simulink model "HCO"  (R2023b)
settings: Solver=VariableStepAuto  StartTime=0.0  StopTime=1  RelTol=1e-3
libraries: simulink x2
settings Model: Creator=Dayan-pc  LastModifiedBy=Dayan-pc
settings OptimizationCC: ReuseModelBlockBuffer=off

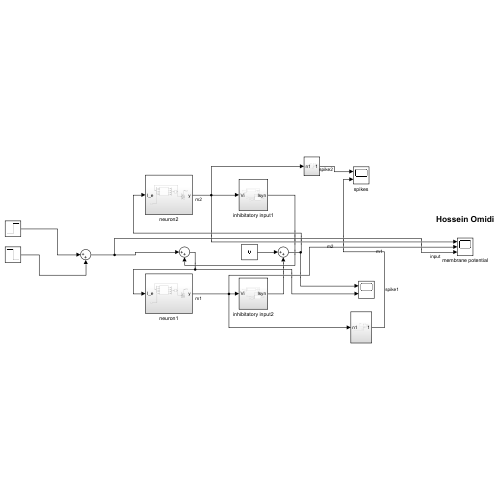
[thumbnail: Simulink's stored preview of the top-level diagram]
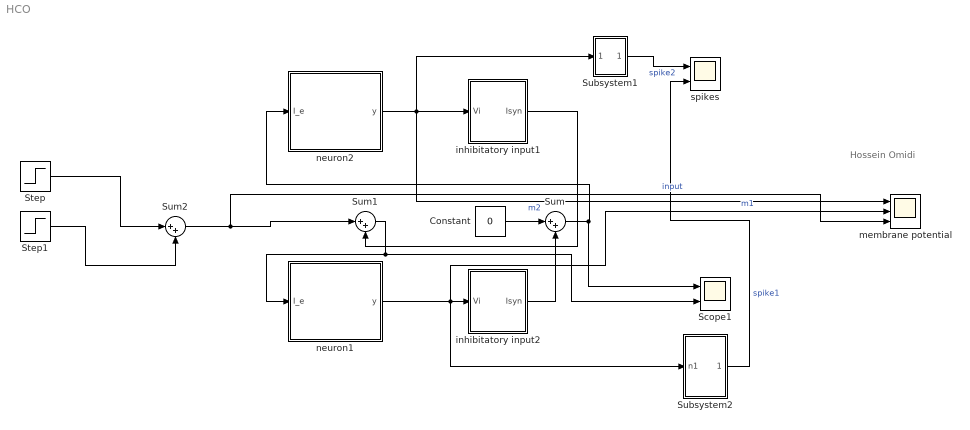
== system HCO ==
  note: Hossein Omidi
  Constant : Constant  Value=0
  Scope1 : Scope  NumInputPorts=2
  Step : Step  Time=.3  After=10  SampleTime=0
  Step1 : Step  Time=.31  After=-10  SampleTime=0
  Subsystem1 : Subsystem
  Subsystem2 : Subsystem
  Sum : Sum  Inputs=|++
  Sum1 : Sum  Inputs=|++
  Sum2 : Sum  Inputs=|++
  inhibitatory input1 : Subsystem
  inhibitatory input2 : Subsystem
  membrane potential : Scope  NumInputPorts=3
  neuron1 : Subsystem
  neuron2 : Subsystem
  spikes : Scope  NumInputPorts=2
  wires:
  neuron2/1(y) -> Subsystem1/1(n1), membrane potential/1, inhibitatory input1/1(Vi)  "m2"
  neuron1/1(y) -> Subsystem2/1(n1), membrane potential/2, inhibitatory input2/1(Vi)  "m1"
  inhibitatory input2/1(Isyn) -> Sum/2
  Sum/1 -> Scope1/1, neuron2/1(I_e)
  Sum1/1 -> Scope1/2, neuron1/1(I_e)
  inhibitatory input1/1(Isyn) -> Sum1/2
  Sum2/1 -> membrane potential/3, Sum1/1  "input"
  Step1/1 -> Sum2/2
  Step/1 -> Sum2/1
  Constant/1 -> Sum/1
  Subsystem1/1(Out1) -> spikes/1  "spike2"
  Subsystem2/1(Out1) -> spikes/2  "spike1"

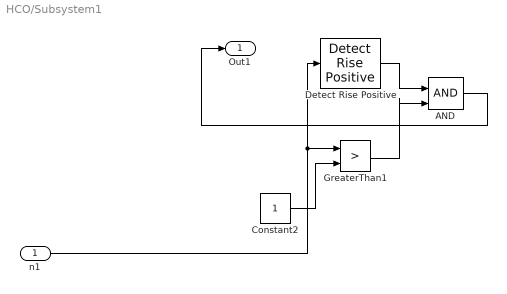
== system HCO/Subsystem1 ==
  n1 : Inport
  AND : Logic  IconShape=distinctive  AllPortsSameDT=off  OutDataTypeStr=boolean
  Constant2 : Constant
  Detect Rise Positive : simulink/Logic and Bit Operations/Detect Rise Positive  vinit=0  OutDataTypeStr=boolean
  GreaterThan1 : RelationalOperator  Operator=>  OutDataTypeStr=boolean  RndMeth=Simplest  InputSameDT=off
  Out1 : Outport
  wires:
  GreaterThan1/1 -> AND/2
  Detect Rise Positive/1 -> AND/1
  Constant2/1 -> GreaterThan1/2
  n1/1 -> GreaterThan1/1, Detect Rise Positive/1
  AND/1 -> Out1/1

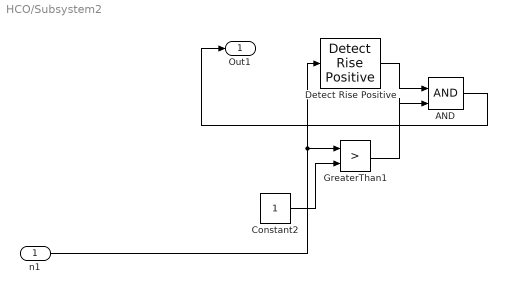
== system HCO/Subsystem2 ==
  n1 : Inport
  AND : Logic  IconShape=distinctive  AllPortsSameDT=off  OutDataTypeStr=boolean
  Constant2 : Constant
  Detect Rise Positive : simulink/Logic and Bit Operations/Detect Rise Positive  vinit=0  OutDataTypeStr=boolean
  GreaterThan1 : RelationalOperator  Operator=>  OutDataTypeStr=boolean  RndMeth=Simplest  InputSameDT=off
  Out1 : Outport
  wires:
  AND/1 -> Out1/1
  n1/1 -> Detect Rise Positive/1, GreaterThan1/1
  Constant2/1 -> GreaterThan1/2
  Detect Rise Positive/1 -> AND/1
  GreaterThan1/1 -> AND/2

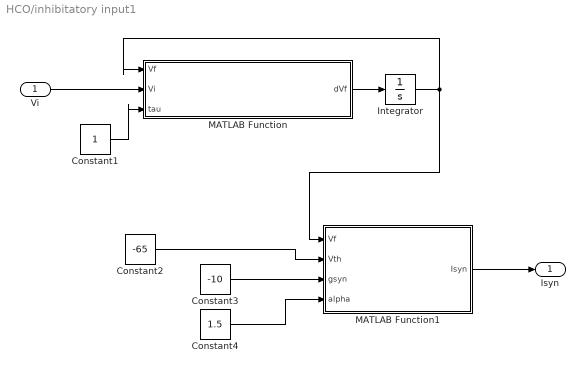
== system HCO/inhibitatory input1 ==
  Vi : Inport
  Constant1 : Constant
  Constant2 : Constant  Value=-65
  Constant3 : Constant  Value=-10
  Constant4 : Constant  Value=1.5
  Integrator : Integrator
  MATLAB Function : MATLAB Function  TreatAsAtomicUnit=on
  MATLAB Function1 : MATLAB Function  TreatAsAtomicUnit=on
  Isyn : Outport
  wires:
  MATLAB Function1/1(Isyn) -> Isyn/1
  Constant1/1 -> MATLAB Function/3(tau)
  Constant4/1 -> MATLAB Function1/4(alpha)
  MATLAB Function/1(dVf) -> Integrator/1
  Integrator/1 -> MATLAB Function1/1(Vf), MATLAB Function/1(Vf)
  Vi/1 -> MATLAB Function/2(Vi)
  Constant3/1 -> MATLAB Function1/3(gsyn)
  Constant2/1 -> MATLAB Function1/2(Vth)

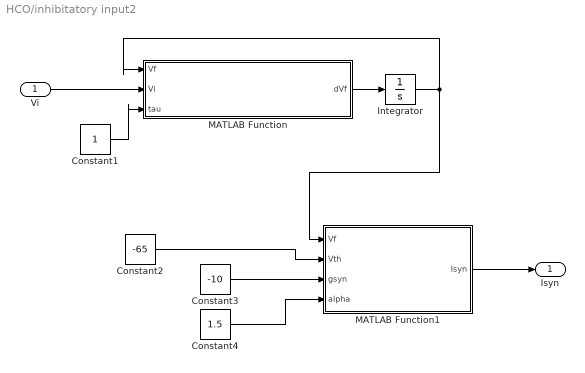
== system HCO/inhibitatory input2 ==
  Vi : Inport
  Constant1 : Constant
  Constant2 : Constant  Value=-65
  Constant3 : Constant  Value=-10
  Constant4 : Constant  Value=1.5
  Integrator : Integrator
  MATLAB Function : MATLAB Function  TreatAsAtomicUnit=on
  MATLAB Function1 : MATLAB Function  TreatAsAtomicUnit=on
  Isyn : Outport
  wires:
  Constant2/1 -> MATLAB Function1/2(Vth)
  Constant3/1 -> MATLAB Function1/3(gsyn)
  Vi/1 -> MATLAB Function/2(Vi)
  Integrator/1 -> MATLAB Function/1(Vf), MATLAB Function1/1(Vf)
  MATLAB Function/1(dVf) -> Integrator/1
  Constant4/1 -> MATLAB Function1/4(alpha)
  Constant1/1 -> MATLAB Function/3(tau)
  MATLAB Function1/1(Isyn) -> Isyn/1

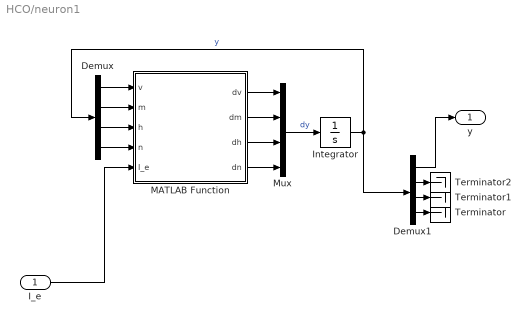
== system HCO/neuron1 ==
  I_e : Inport
  Demux : Demux
  Demux1 : Demux
  Integrator : Integrator  InitialCondition=[-65; 0.05; 0.60; 0.32]
  MATLAB Function : MATLAB Function  TreatAsAtomicUnit=on
  Mux : Mux
  Terminator : Terminator
  Terminator1 : Terminator
  Terminator2 : Terminator
  y : Outport
  wires:
  Demux1/1 -> y/1
  Demux1/2 -> Terminator2/1
  Demux1/3 -> Terminator1/1
  Demux1/4 -> Terminator/1
  I_e/1 -> MATLAB Function/5(I_e)
  MATLAB Function/2(dm) -> Mux/2
  Demux/4 -> MATLAB Function/4(n)
  Demux/2 -> MATLAB Function/2(m)
  Demux/3 -> MATLAB Function/3(h)
  Integrator/1 -> Demux1/1, Demux/1  "y"
  MATLAB Function/4(dn) -> Mux/4
  MATLAB Function/3(dh) -> Mux/3
  Demux/1 -> MATLAB Function/1(v)
  Mux/1 -> Integrator/1  "dy"
  MATLAB Function/1(dv) -> Mux/1

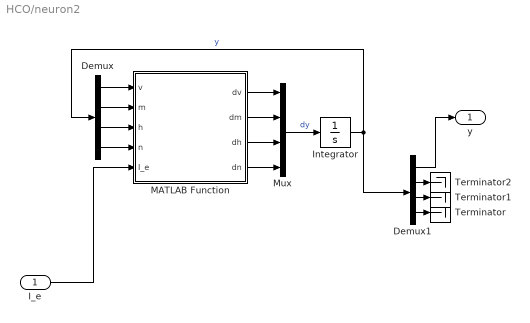
== system HCO/neuron2 ==
  I_e : Inport
  Demux : Demux
  Demux1 : Demux
  Integrator : Integrator  InitialCondition=[-65; 0.05; 0.60; 0.32]
  MATLAB Function : MATLAB Function  TreatAsAtomicUnit=on
  Mux : Mux
  Terminator : Terminator
  Terminator1 : Terminator
  Terminator2 : Terminator
  y : Outport
  wires:
  MATLAB Function/1(dv) -> Mux/1
  Mux/1 -> Integrator/1  "dy"
  Demux/1 -> MATLAB Function/1(v)
  MATLAB Function/3(dh) -> Mux/3
  MATLAB Function/4(dn) -> Mux/4
  Integrator/1 -> Demux/1, Demux1/1  "y"
  Demux/3 -> MATLAB Function/3(h)
  Demux/2 -> MATLAB Function/2(m)
  Demux/4 -> MATLAB Function/4(n)
  MATLAB Function/2(dm) -> Mux/2
  I_e/1 -> MATLAB Function/5(I_e)
  Demux1/4 -> Terminator/1
  Demux1/3 -> Terminator1/1
  Demux1/2 -> Terminator2/1
  Demux1/1 -> y/1

== matlab function HCO/inhibitatory input2/MATLAB Function ==
  data: Vf input; dVf output; Vi input; tau input
function dVf = synapse_filter_deriv(Vf, Vi, tau)
% ODE for the synaptic low-pass filter state Vf
% tau * dVf/dt = Vpre - Vf  ->  dVf/dt = (Vpre - Vf)/tau
% Inputs:
%   Vf   - current filter state (mV)
%   Vpre - presynaptic membrane voltage (mV)
%   tau  - filter time constant (ms, >0)
% Output:
%   dVf  - time derivative of Vf (mV/ms)

% numeric safety

dVf = 1000*(Vi - Vf) / tau;
end

== matlab function HCO/neuron2/MATLAB Function ==
  data: v input; dv output; m input; h input; n input; I_e input; dm output; dh output; dn output
function [dv, dm, dh, dn] = hh_block(v, m, h, n, I_e)
% HH ODEs for Simulink MATLAB Function block
% Inputs: v,m,h,n (states), I_e total injected current (uA/cm^2)
% Outputs: dv,dm,dh,dn (state derivatives)

    % Params
    C_m = 1.0; gNa = 120.0; gK = 36.0; gL = 0.3;
    ENa = 50.0; EK = -77.0; EL = -54.387;

    % Safe division
    am_num = 0.1 * (v + 40.0);
    am_den = 1.0 - exp(-(v + 40.0)/10.0);
    %if abs(am_den) < epsd, am_den = sign(am_den)*epsd + (am_den==0)*epsd; end
    alpha_m = am_num / am_den;

    beta_m = 4.0 * exp(-(v + 65.0)/18.0);
    alpha_h = 0.07 * exp(-(v + 65.0)/20.0);
    beta_h  = 1.0 / (1.0 + exp(-(v + 35.0)/10.0));

    an_num = 0.01 * (v + 55.0);
    an_den = 1.0 - exp(-(v + 55.0)/10.0);
    %if abs(an_den) < epsd, an_den = sign(an_den)*epsd + (an_den==0)*epsd; end
    alpha_n = an_num / an_den;

    beta_n = 0.125 * exp(-(v + 65.0)/80.0);

    % x_inf and tau
    denom_m = alpha_m + beta_m; 
    denom_h = alpha_h + beta_h; 
    denom_n = alpha_n + beta_n;

    m_inf = alpha_m / denom_m; tau_m = 1.0 / denom_m;
    h_inf = alpha_h / denom_h; tau_h = 1.0 / denom_h;
    n_inf = alpha_n / denom_n; tau_n = 1.0 / denom_n;

    % Currents
    I_Na = gNa * (m^3) * h * (v - ENa);
    I_K  = gK  * (n^4) * (v - EK);
    I_L  = gL  * (v - EL);

    % ODEs
    dv = 1000*(-I_L - I_Na - I_K + I_e) / C_m;
    dm = 1000*(m_inf - m) / tau_m;
    dh = 1000*(h_inf - h) / tau_h;
    dn = 1000*(n_inf - n) / tau_n;
end

== matlab function HCO/inhibitatory input2/MATLAB Function1 ==
  data: Vf input; Isyn output; Vth input; gsyn input; alpha input
function Isyn = synapse_current(Vf, Vth, gsyn, alpha)
% Current-based synapse (paper's model)
% Isyn = gsyn / (1 + exp(-alpha*(Vf - Vth)))
% Inputs:
%   Vf    - filtered presynaptic voltage (mV)
%   Vth   - threshold (mV)
%   gsyn  - synaptic strength (uA/cm^2). >0 excitatory, <0 inhibitory
%   alpha - sigmoid slope (>0)
% Output:
%   Isyn  - synaptic current to inject into postsynaptic neuron (uA/cm^2)



% Synapse nonlinearity (paper)
s = Vf - Vth;                % onto neuron 2
Isyn = gsyn / (1 + exp(-alpha * s));
end

== matlab function HCO/neuron1/MATLAB Function ==
  data: v input; dv output; m input; h input; n input; I_e input; dm output; dh output; dn output
function [dv, dm, dh, dn] = hh_block(v, m, h, n, I_e)
% HH ODEs for Simulink MATLAB Function block
% Inputs: v,m,h,n (states), I_e total injected current (uA/cm^2)
% Outputs: dv,dm,dh,dn (state derivatives)

    % Params
    C_m = 1.0; gNa = 120.0; gK = 36.0; gL = 0.3;
    ENa = 50.0; EK = -77.0; EL = -54.387;

    % Safe division
    am_num = 0.1 * (v + 40.0);
    am_den = 1.0 - exp(-(v + 40.0)/10.0);
    %if abs(am_den) < epsd, am_den = sign(am_den)*epsd + (am_den==0)*epsd; end
    alpha_m = am_num / am_den;

    beta_m = 4.0 * exp(-(v + 65.0)/18.0);
    alpha_h = 0.07 * exp(-(v + 65.0)/20.0);
    beta_h  = 1.0 / (1.0 + exp(-(v + 35.0)/10.0));

    an_num = 0.01 * (v + 55.0);
    an_den = 1.0 - exp(-(v + 55.0)/10.0);
    %if abs(an_den) < epsd, an_den = sign(an_den)*epsd + (an_den==0)*epsd; end
    alpha_n = an_num / an_den;

    beta_n = 0.125 * exp(-(v + 65.0)/80.0);

    % x_inf and tau
    denom_m = alpha_m + beta_m; 
    denom_h = alpha_h + beta_h; 
    denom_n = alpha_n + beta_n;

    m_inf = alpha_m / denom_m; tau_m = 1.0 / denom_m;
    h_inf = alpha_h / denom_h; tau_h = 1.0 / denom_h;
    n_inf = alpha_n / denom_n; tau_n = 1.0 / denom_n;

    % Currents
    I_Na = gNa * (m^3) * h * (v - ENa);
    I_K  = gK  * (n^4) * (v - EK);
    I_L  = gL  * (v - EL);

    % ODEs
    dv = 1000*(-I_L - I_Na - I_K + I_e) / C_m;
    dm = 1000*(m_inf - m) / tau_m;
    dh = 1000*(h_inf - h) / tau_h;
    dn = 1000*(n_inf - n) / tau_n;
end

== matlab function HCO/inhibitatory input1/MATLAB Function ==
  data: Vf input; dVf output; Vi input; tau input
function dVf = synapse_filter_deriv(Vf, Vi, tau)
% ODE for the synaptic low-pass filter state Vf
% tau * dVf/dt = Vpre - Vf  ->  dVf/dt = (Vpre - Vf)/tau
% Inputs:
%   Vf   - current filter state (mV)
%   Vpre - presynaptic membrane voltage (mV)
%   tau  - filter time constant (ms, >0)
% Output:
%   dVf  - time derivative of Vf (mV/ms)

% numeric safety

dVf = 1000*(Vi - Vf) / tau;
end

== matlab function HCO/inhibitatory input1/MATLAB Function1 ==
  data: Vf input; Isyn output; Vth input; gsyn input; alpha input
function Isyn = synapse_current(Vf, Vth, gsyn, alpha)
% Current-based synapse (paper's model)
% Isyn = gsyn / (1 + exp(-alpha*(Vf - Vth)))
% Inputs:
%   Vf    - filtered presynaptic voltage (mV)
%   Vth   - threshold (mV)
%   gsyn  - synaptic strength (uA/cm^2). >0 excitatory, <0 inhibitory
%   alpha - sigmoid slope (>0)
% Output:
%   Isyn  - synaptic current to inject into postsynaptic neuron (uA/cm^2)



% Synapse nonlinearity (paper)
s = Vf - Vth;                % onto neuron 2
Isyn = gsyn / (1 + exp(-alpha * s));
end
